simulink model "DivideNConquer"  (R2023a)
settings: Solver=VariableStepAuto  StartTime=0  StopTime=6012  MinStep=1e-2  RelTol=1e-3  AbsTol=1e-9
model workspace (MAT data in the model file):
  Cap = 4
  Grade = 0
  QHbatt = 70
  QLbatt = 40
  Trqmax = 400
  Vref = 650
values from neighbouring files (symbols this model uses):
  s = (id-1)*n_sim + 1    [LHSdesign.m]
undefined symbols (not defined in the file or in its folder): Qbatt, Vbatt
libraries: fl_lib x29, nesl_utility x15, sdl_lib x9, ee_lib x7, batteryecm_lib x1, autolibshared x1, slpidlib x1
(part 1 of 2)
settings Model: Creator=luiz4  LastModifiedBy=NUC04
settings SolverCC: MaxConsecutiveZCs=10000  MaxConsecutiveMinStep=12  ZeroCrossControl=EnableAll  ZeroCrossAlgorithm=Adaptive  EnableFixedStepZeroCrossing=on
settings OptimizationCC: ReuseModelBlockBuffer=off

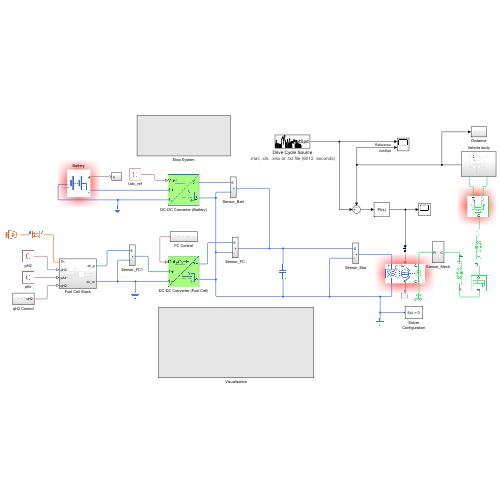
[thumbnail: Simulink's stored preview of the top-level diagram]
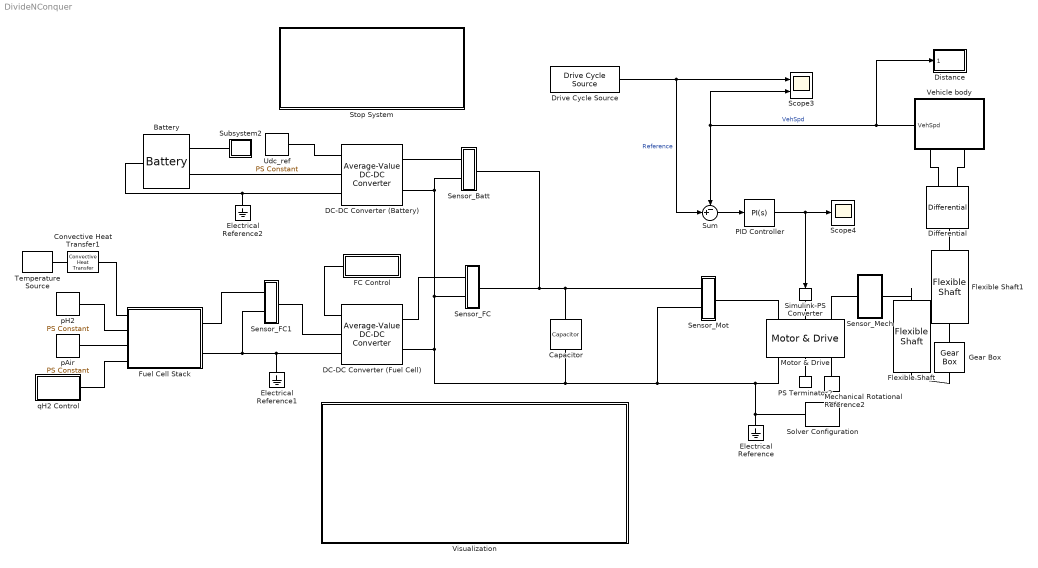
== system DivideNConquer ==
  Battery : batteryecm_lib/Battery  Vnom=Vbatt V  prm_dir=simscape.enum.battery.prm_dir.enabled  R1_dis=0.05 Ohm  R1_ch=0.05 Ohm  R1=0.05 Ohm  prm_AH=2  AH=Qbatt hr*A  V1=(4/5)*Vbatt V  AH1=0.5*Qbatt hr*A  prm_R2=1  R2=2000 Ohm  Tmeas=343.15 K  charge_measurement_port=simscape.enum.battery.enable.yes  prm_dyn=1  Rp1=0.005 Ohm  tau1=30 s  Rp2=0.005 Ohm  tau2=30 s  Rp3=0.005 Ohm  tau3=30 s  Rp4=0.005 Ohm  tau4=30 s  Rp5=0.005 Ohm  tau5=30 s  prm_fade=1  N_fade=100  AH_fade=45 hr*A  R1_fade=2.02 Ohm  R1_ch_fade=2.02 Ohm  V1_fade=10.35 V  prm_age=1  prm_age_OCV=1  OCV_age=0.9  SOC_age=60  Tmeas_age=298.15 K  delta_time_age_vec=[0] d  temperature_age_vec=[273] K  OCV_scaling_age=2.2134e6  OCV_offset_age=1.632e6  temp_exp_age=0.515833569 V  t_exp_age=0.75  Vnom_T2=12 V  R1_T2=2.2 Ohm  R1_T2_dis=2.2 Ohm  R1_T2_ch=2.2 Ohm  V1_T2=11.4 V  R2_T2=2200 Ohm  Rp1_T2=0.005 Ohm  tau1_T2=30 s  Rp2_T2=0.005 Ohm  tau2_T2=30 s  Rp3_T2=0.005 Ohm  tau3_T2=30 s  Rp4_T2=0.005 Ohm  tau4_T2=30 s  Rp5_T2=0.005 Ohm  tau5_T2=30 s  Tmeas2=273.15 K  thermal_port=simscape.enum.thermaleffects.omit  thermal_mass=30000 J/K  i_specify=off  i_priority=None  i=0 A  i_nominal_specify=off  i_nominal_unit=A  i_nominal_value=1  v_specify=on  v_priority=High  v=Vbatt V  v_nominal_specify=off  v_nominal_unit=V  v_nominal_value=1  charge_specify=on  charge_priority=High  charge=QHbatt*Qbatt/100 hr*A  charge_nominal_specify=off  charge_nominal_unit=A*hr  charge_nominal_value=1  num_cycles_specify=off  num_cycles_priority=High  num_cycles=0  num_cycles_nominal_specify=off  num_cycles_nominal_unit=1  num_cycles_nominal_value=1  temperature_specify=off  temperature_priority=High  temperature=298.15 K  temperature_nominal_specify=off  temperature_nominal_unit=K  temperature_nominal_value=1
      settings: LogSimulationData=on  InternalSimscapePortConfiguration="{\"Bottom\":[],\"Left\":[{\"id\":\"p\",\"label\":\"+\",\"type\":\"foundation.electrical.electrical\"},{\"id\":\"q\",\"label\":\"q\",\"type\":\"output\"}],\"Right\":[{\"id\":\"n\",\"label\":\"-\",\"type\":\"foundation.electrical.electrical\"}],\"Top\":[]}"
  Capacitor : fl_lib/Electrical/Electrical Elements/Capacitor  c=Cap F  r=1e-6 Ohm  g=0 1/Ohm  i_specify=off  i_priority=None  i=0 A  i_nominal_specify=off  i_nominal_unit=A  i_nominal_value=1  v_specify=off  v_priority=None  v=0 V  v_nominal_specify=off  v_nominal_unit=V  v_nominal_value=1  vc_specify=on  vc_priority=High  vc=0 V  vc_nominal_specify=on  vc_nominal_unit=V  vc_nominal_value=Vref
  Convective Heat Transfer1 : fl_lib/Thermal/Thermal Elements/Convective Heat Transfer  thermal_type=foundation.enum.constant_variable.constant  area=300 cm^2  heat_tr_coeff=75 W/(m^2 * K)  min_heat_tr_coeff=1e-3 W/(K*m^2)  T_specify=off  T_priority=None  T=0 K  T_nominal_specify=off  T_nominal_unit=K  T_nominal_value=1  Q_specify=off  Q_priority=None  Q=0 W  Q_nominal_specify=off  Q_nominal_unit=W  Q_nominal_value=1
  DC-DC Converter (Battery) : ee_lib/Semiconductors & Converters/Converters/Average-Value DC-DC Converter  control_option=ee.enum.converters.controlinput.voltage  converter_type=ee.enum.converters.dcdctype.boost  efficiency_option=ee.enum.converters.efficiency.constant  efficiency_fixed=90  i_vec=[0, 2, 5] A  efficiency_vec=[90, 95, 98]
      settings: LogSimulationData=on  InternalSimscapePortConfiguration="{\"Bottom\":[],\"Left\":[{\"id\":\"Vref\",\"label\":\"Vref\",\"type\":\"input\"},{\"id\":\"p1\",\"label\":\"1+\",\"type\":\"foundation.electrical.electrical\"},{\"id\":\"n1\",\"label\":\"1-\",\"type\":\"foundation.electrical.electrical\"}],\"Right\":[{\"id\":\"p2\",\"label\":\"2+\",\"type\":\"foundation.electrical.electrical\"},{\"id\":\"n2\",\"label\":\"2-\",\"type\":\"foundation.electrical.electrical\"}],\"Top\":[]}"
  DC-DC Converter (Fuel Cell) : ee_lib/Semiconductors & Converters/Converters/Average-Value DC-DC Converter  control_option=ee.enum.converters.controlinput.dutycycle  converter_type=ee.enum.converters.dcdctype.boost  efficiency_option=ee.enum.converters.efficiency.constant  efficiency_fixed=90  i_vec=[0, 2, 5] A  efficiency_vec=[90, 95, 98]
      settings: LogSimulationData=on  InternalSimscapePortConfiguration="{\"Bottom\":[],\"Left\":[{\"id\":\"DutyCycle\",\"label\":\"DutyCycle\",\"type\":\"input\"},{\"id\":\"p1\",\"label\":\"1+\",\"type\":\"foundation.electrical.electrical\"},{\"id\":\"n1\",\"label\":\"1-\",\"type\":\"foundation.electrical.electrical\"}],\"Right\":[{\"id\":\"p2\",\"label\":\"2+\",\"type\":\"foundation.electrical.electrical\"},{\"id\":\"n2\",\"label\":\"2-\",\"type\":\"foundation.electrical.electrical\"}],\"Top\":[]}"
  Differential : sdl_lib/Gears/Differential  driveshaft_location=sdl.enum.differential_orientation.right  cd_ratio=Rdiff  friction_model=sdl.enum.gear_friction.none  efficiency=[.85, .92]  temperature_TLU=[280, 300, 320] K  efficiency_ss_TLU=[.95, .9, .85]  efficiency_cd_TLU=[.95, .9, .85]  pwr_thr=[.001, .001] W  mu_visc=[0, 0] N*m*s/rad  model_inertia=simscape.enum.onoff.on  carrier_inertia=0.001 kg*m^2  planet_inertia=0.001 kg*m^2  thermal_mass=50 J/K  T_init=300 K
  Distance : Subsystem
  Drive Cycle Source : autolibshared/Drive Cycle Source  cycleVar=.mat, .xls, .xlsx or .txt file  wsVar=DriveCycle  fileVar=cycleMASTER.mat  tfinal="6012  seconds"  cycleRepeat=off  outAccPort=off  outGearPort=off  gearList=No gear data  t_wot1=5  xdot_woto=0  xdot_wot1=30  t_wot2=20  xdot_wot2=0  t_wotend=30  srcUnit=m/s  outUnit=m/s  srcAccUnit=m/s/s  outAccUnit=m/s^2  dt=0  aMode=1  faultOption=off  velBnd=2  velBndUnit=mph  inUnit=m/s  timeBnd=1  failOption=off  stopSim=off  maxFaultCnt=10  maxFaultTime=2  maxTotFaultTime=15  traceOption=off  dtTrace=1  traceWindow=10  lastDCname=Custom Data Set 1  lastOutUnit=mph  lastDT=0  lastTB=1  lastSB=2  forceCalcBound=off
  Electrical Reference : fl_lib/Electrical/Electrical Elements/Electrical Reference
  Electrical Reference1 : fl_lib/Electrical/Electrical Elements/Electrical Reference
  Electrical Reference2 : fl_lib/Electrical/Electrical Elements/Electrical Reference
  FC Control : Subsystem
  Flexible Shaft : sdl_lib/Couplings & Drives/Flexible Shaft  modelTorsion=true  modelTransverse=false  n_segments=1  parameterization=sdl.enum.shaftParameterization.StiffnessInertia  length=1 m  lengths=[1, .5, .25] m  shaft_stiffness=1e5 N*m/rad  shaft_inertia=0.1 kg*m^2  shaft_stiffnesses=[400000, 200000, 100000] N*m/rad  shaft_inertias=[.025, .02, .015] kg*m^2  eiIN=5e5 Pa*m^4  rhoaIN=19 kg/m  eiINs=[600000, 500000, 400000] Pa*m^4  rhoaINs=[20, 19, 18] kg/m  density=7.8e3 kg/m^3  shear_modulus=7.93e9 Pa  elastic_modulus=200e9 Pa  shaft_construction=sdl.enum.shaftConstruction.solid  diameter_outer=0.075 m  diameter_inner=0.05 m  diameter_outers=[.085, .075, .065] m  diameter_inners=[.055, .05, .045] m  damping_ratio=0.001  mu_visc_BF=[0, 0] N*m*s/rad  mu_visc=[0, 0] N*m*s/rad  initial_deflection=0 rad  initial_velocity=0 rpm  num_supports=sdl.enum.num_supports.two  z_support=[0, 1] m  boundaryB1=sdl.enum.shaftSupport.clamp  DrotB1_row=[1000, 1000] N*m*s/rad  DtransB1_row=[20000, -44000, -44000, 350000] N*s/m  DtransB1_w_mat=[20000, -44000, -44000, 350000; 10000, -25000, -25000, 140000; 5000, -10000, -10000, 20000] N*s/m  KrotB1_row=[10000, 10000] N*m/rad  KtransB1_row=[1000000, -200000, -300000, 5000000] N/m  KtransB1_w_mat=[1000000, -600000, -3500000, 8000000; 1000000, -200000, -3000000, 5000000; 1000000, -50000, -2500000, 3000000] N/m  boundaryI1=sdl.enum.shaftSupport.clamp  DrotI1_row=[1000, 1000] N*m*s/rad  DtransI1_row=[20000, -44000, -44000, 350000] N*s/m  DtransI1_w_mat=[20000, -44000, -44000, 350000; 10000, -25000, -25000, 140000; 5000, -10000, -10000, 20000] N*s/m  KrotI1_row=[10000, 10000] N*m/rad  KtransI1_row=[1000000, -200000, -300000, 5000000] N/m  KtransI1_w_mat=[1000000, -600000, -3500000, 8000000; 1000000, -200000, -3000000, 5000000; 1000000, -50000, -2500000, 3000000] N/m  boundaryI2=sdl.enum.shaftSupport.clamp  DrotI2_row=[1000, 1000] N*m*s/rad  DtransI2_row=[20000, -44000, -44000, 350000] N*s/m  DtransI2_w_mat=[20000, -44000, -44000, 350000; 10000, -25000, -25000, 140000; 5000, -10000, -10000, 20000] N*s/m  KrotI2_row=[10000, 10000] N*m/rad  KtransI2_row=[1000000, -200000, -300000, 5000000] N/m  KtransI2_w_mat=[1000000, -600000, -3500000, 8000000; 1000000, -200000, -3000000, 5000000; 1000000, -50000, -2500000, 3000000] N/m  boundaryF1=sdl.enum.shaftSupport.clamp  DrotF1_row=[1000, 1000] N*m*s/rad  DtransF1_row=[20000, -44000, -44000, 350000] N*s/m  DtransF1_w_mat=[20000, -44000, -44000, 350000; 10000, -25000, -25000, 140000; 5000, -10000, -10000, 20000] N*s/m  KrotF1_row=[10000, 10000] N*m/rad  KtransF1_row=[1000000, -200000, -300000, 5000000] N/m  KtransF1_w_mat=[1000000, -600000, -3500000, 8000000; 1000000, -200000, -3000000, 5000000; 1000000, -50000, -2500000, 3000000] N/m  bearing_speed=[200, 500, 1500] rpm  alpha=10 1/s  beta=1e-8 s  noDisk=sdl.enum.shaftDisks.none  zDisk=0.5 m  mDiskIN=2 kg  IdDiskIN=0.025 kg*m^2  IpDiskIN=0.050 kg*m^2  enable_static_unbalance=true  offsetMR=[.01, .01] kg*m  offsetMR_initialAngleIN=[0, pi] rad  offsetMassLocation=[.33, .67] m  enable_external_force=false  externalForce=[1, 2] N  externalForceHarmonic=[.5, 2]  externalLoadAngle=[pi / 2, 3 * pi / 4] rad  zExternalLoad=[.25, .75] m  AnalysisMethod=sdl.enum.bendingAnalysisMethod.LumpedMass  ModeInputMethod=sdl.enum.modeInputMethod.SimscapeDetermined  numModesIn=6  mode_speed_dependency=sdl.enum.mode_speed_dependency.Static  OmegaNom=5000 rpm  wMax=1e8 rpm  dz=0.01 m  userMode_w=[280, 644, 615, 1285] rad/s  userMode_w_mat=[257, 780, 580, 1560; 280, 644, 615, 1285; 294, 513, 636, 1020] rad/s  userMode_z=[0, .1, .2, .3, .4, .5, .6, .7, .8, .9, 1] m  userMode_shapeX=[.1648, .0086, -.2759, .0162; .1671, .0093, -.2231, .0133; .1691, .01, -.1689, .0102; .1707, .0105, -.1135, .007; .1717, .0108, -.057, .0035; .1721, .0109, 0, 0; .1717, .0108, .057, -.0035; .1707, .0105, .1135, -.007; .1691, .01, .1689, -.0102; .1671, .0093, .2231, -.0133; .1648, .0086, .2759, -.0162]  userMode_shapeX_mat=cat(3, [.1842, .0134, -.3072, .0272; .1863, .0152, -.2482, .0226; .1882, .0169, -.1878, .0176; .1897, .0182, -.1261, .0121; .1906, .019, -.0634, .0062; .191, .0193, 0, 0; .1906, .019, .0634, -.0062; .1897, .0182, .1261, -.0121; .1882, .0169, .1878, -.0176; .1863, .0152, .2482, -.0226; .1842, .0134, .3072, -.0272], [.1648, .0086, -.2759, .0162; .1671, .0093, -.2231, .0133; .1691, .01, -.1689, .0102; .1707, .0105, -.1135, .007; .1717, .0108, -.057, .0035; .1721, .0109, 0, 0; .1717, .0108, .057, -.0035; .1707, .0105, .1135, -.007; .1691, .01, .1689, -.0102; .1671, .0093, .2231, -.0133; .1648, .0086, .2759, -.0162], [.1291, .0046, -.2166, .0082; .131, .0048, -.1751, .0067; .1327, .005, -.1327, .0051; .1341, .0052, -.0891, .0035; .135, .0053, -.0448, .0017; .1353, .0053, 0, 0; .135, .0053, .0448, -.0017; .1341, .0052, .0891, -.0035; .1327, .005, .1327, -.0051; .131, .0048, .1751, -.0067; .1291, .0046, .2166, -.0082])  userMode_shapeY=[.1193, -.1784, -.1997, -.3348; .1209, -.1933, -.1615, -.2751; .1224, -.2068, -.1223, -.2119; .1235, -.2176, -.0821, -.1445; .1243, -.2245, -.0413, -.0734; .1246, -.2269, 0, 0; .1243, -.2245, .0413, .0734; .1235, -.2176, .0821, .1445; .1224, -.2068, .1223, .2119; .1209, -.1933, .1615, .2751; .1193, -.1784, .1997, .3348]  userMode_shapeY_mat=cat(3, [.0885, -.1625, -.1475, -.3301; .0895, -.1847, -.1192, -.2745; .0904, -.2048, -.0902, -.2141; .0911, -.2209, -.0606, -.1475; .0916, -.2313, -.0304, -.0754; .0917, -.2349, 0, 0; .0916, -.2313, .0304, .0754; .0911, -.2209, .0606, .1475; .0904, -.2048, .0902, .2141; .0895, -.1847, .1192, .2745; .0885, -.1625, .1475, .3301], [.1193, -.1784, -.1997, -.3348; .1209, -.1933, -.1615, -.2751; .1224, -.2068, -.1223, -.2119; .1235, -.2176, -.0821, -.1445; .1243, -.2245, -.0413, -.0734; .1246, -.2269, 0, 0; .1243, -.2245, .0413, .0734; .1235, -.2176, .0821, .1445; .1224, -.2068, .1223, .2119; .1209, -.1933, .1615, .2751; .1193, -.1784, .1997, .3348], [.1566, -.1901, -.2628, -.3377; .1589, -.1994, -.2125, -.2753; .161, -.2079, -.1609, -.2103; .1627, -.2146, -.1081, -.1424; .1638, -.219, -.0544, -.0719; .1642, -.2205, 0, 0; .1638, -.219, .0544, .0719; .1627, -.2146, .1081, .1424; .161, -.2079, .1609, .2103; .1589, -.1994, .2125, .2753; .1566, -.1901, .2628, .3377])  eta_lumped_nominal=1  etaDer_lumped_nominal=1  eta_modal_nominal=1  etaDer_modal_nominal=1
      settings: InternalSimscapePortConfiguration="{\"Bottom\":[],\"Left\":[{\"id\":\"B\",\"label\":\"B\",\"type\":\"foundation.mechanical.rotational.rotational\"}],\"Right\":[{\"id\":\"F\",\"label\":\"F\",\"type\":\"foundation.mechanical.rotational.rotational\"}],\"Top\":[]}"
  Flexible Shaft1 : sdl_lib/Couplings & Drives/Flexible Shaft  modelTorsion=true  modelTransverse=false  n_segments=1  parameterization=sdl.enum.shaftParameterization.StiffnessInertia  length=1 m  lengths=[1, .5, .25] m  shaft_stiffness=1e5 N*m/rad  shaft_inertia=0.1 kg*m^2  shaft_stiffnesses=[400000, 200000, 100000] N*m/rad  shaft_inertias=[.025, .02, .015] kg*m^2  eiIN=5e5 Pa*m^4  rhoaIN=19 kg/m  eiINs=[600000, 500000, 400000] Pa*m^4  rhoaINs=[20, 19, 18] kg/m  density=7.8e3 kg/m^3  shear_modulus=7.93e9 Pa  elastic_modulus=200e9 Pa  shaft_construction=sdl.enum.shaftConstruction.solid  diameter_outer=0.075 m  diameter_inner=0.05 m  diameter_outers=[.085, .075, .065] m  diameter_inners=[.055, .05, .045] m  damping_ratio=0.001  mu_visc_BF=[0, 0] N*m*s/rad  mu_visc=[0, 0] N*m*s/rad  initial_deflection=0 rad  initial_velocity=0 rpm  num_supports=sdl.enum.num_supports.two  z_support=[0, 1] m  boundaryB1=sdl.enum.shaftSupport.clamp  DrotB1_row=[1000, 1000] N*m*s/rad  DtransB1_row=[20000, -44000, -44000, 350000] N*s/m  DtransB1_w_mat=[20000, -44000, -44000, 350000; 10000, -25000, -25000, 140000; 5000, -10000, -10000, 20000] N*s/m  KrotB1_row=[10000, 10000] N*m/rad  KtransB1_row=[1000000, -200000, -300000, 5000000] N/m  KtransB1_w_mat=[1000000, -600000, -3500000, 8000000; 1000000, -200000, -3000000, 5000000; 1000000, -50000, -2500000, 3000000] N/m  boundaryI1=sdl.enum.shaftSupport.clamp  DrotI1_row=[1000, 1000] N*m*s/rad  DtransI1_row=[20000, -44000, -44000, 350000] N*s/m  DtransI1_w_mat=[20000, -44000, -44000, 350000; 10000, -25000, -25000, 140000; 5000, -10000, -10000, 20000] N*s/m  KrotI1_row=[10000, 10000] N*m/rad  KtransI1_row=[1000000, -200000, -300000, 5000000] N/m  KtransI1_w_mat=[1000000, -600000, -3500000, 8000000; 1000000, -200000, -3000000, 5000000; 1000000, -50000, -2500000, 3000000] N/m  boundaryI2=sdl.enum.shaftSupport.clamp  DrotI2_row=[1000, 1000] N*m*s/rad  DtransI2_row=[20000, -44000, -44000, 350000] N*s/m  DtransI2_w_mat=[20000, -44000, -44000, 350000; 10000, -25000, -25000, 140000; 5000, -10000, -10000, 20000] N*s/m  KrotI2_row=[10000, 10000] N*m/rad  KtransI2_row=[1000000, -200000, -300000, 5000000] N/m  KtransI2_w_mat=[1000000, -600000, -3500000, 8000000; 1000000, -200000, -3000000, 5000000; 1000000, -50000, -2500000, 3000000] N/m  boundaryF1=sdl.enum.shaftSupport.clamp  DrotF1_row=[1000, 1000] N*m*s/rad  DtransF1_row=[20000, -44000, -44000, 350000] N*s/m  DtransF1_w_mat=[20000, -44000, -44000, 350000; 10000, -25000, -25000, 140000; 5000, -10000, -10000, 20000] N*s/m  KrotF1_row=[10000, 10000] N*m/rad  KtransF1_row=[1000000, -200000, -300000, 5000000] N/m  KtransF1_w_mat=[1000000, -600000, -3500000, 8000000; 1000000, -200000, -3000000, 5000000; 1000000, -50000, -2500000, 3000000] N/m  bearing_speed=[200, 500, 1500] rpm  alpha=10 1/s  beta=1e-8 s  noDisk=sdl.enum.shaftDisks.none  zDisk=0.5 m  mDiskIN=2 kg  IdDiskIN=0.025 kg*m^2  IpDiskIN=0.050 kg*m^2  enable_static_unbalance=true  offsetMR=[.01, .01] kg*m  offsetMR_initialAngleIN=[0, pi] rad  offsetMassLocation=[.33, .67] m  enable_external_force=false  externalForce=[1, 2] N  externalForceHarmonic=[.5, 2]  externalLoadAngle=[pi / 2, 3 * pi / 4] rad  zExternalLoad=[.25, .75] m  AnalysisMethod=sdl.enum.bendingAnalysisMethod.LumpedMass  ModeInputMethod=sdl.enum.modeInputMethod.SimscapeDetermined  numModesIn=6  mode_speed_dependency=sdl.enum.mode_speed_dependency.Static  OmegaNom=5000 rpm  wMax=1e8 rpm  dz=0.01 m  userMode_w=[280, 644, 615, 1285] rad/s  userMode_w_mat=[257, 780, 580, 1560; 280, 644, 615, 1285; 294, 513, 636, 1020] rad/s  userMode_z=[0, .1, .2, .3, .4, .5, .6, .7, .8, .9, 1] m  userMode_shapeX=[.1648, .0086, -.2759, .0162; .1671, .0093, -.2231, .0133; .1691, .01, -.1689, .0102; .1707, .0105, -.1135, .007; .1717, .0108, -.057, .0035; .1721, .0109, 0, 0; .1717, .0108, .057, -.0035; .1707, .0105, .1135, -.007; .1691, .01, .1689, -.0102; .1671, .0093, .2231, -.0133; .1648, .0086, .2759, -.0162]  userMode_shapeX_mat=cat(3, [.1842, .0134, -.3072, .0272; .1863, .0152, -.2482, .0226; .1882, .0169, -.1878, .0176; .1897, .0182, -.1261, .0121; .1906, .019, -.0634, .0062; .191, .0193, 0, 0; .1906, .019, .0634, -.0062; .1897, .0182, .1261, -.0121; .1882, .0169, .1878, -.0176; .1863, .0152, .2482, -.0226; .1842, .0134, .3072, -.0272], [.1648, .0086, -.2759, .0162; .1671, .0093, -.2231, .0133; .1691, .01, -.1689, .0102; .1707, .0105, -.1135, .007; .1717, .0108, -.057, .0035; .1721, .0109, 0, 0; .1717, .0108, .057, -.0035; .1707, .0105, .1135, -.007; .1691, .01, .1689, -.0102; .1671, .0093, .2231, -.0133; .1648, .0086, .2759, -.0162], [.1291, .0046, -.2166, .0082; .131, .0048, -.1751, .0067; .1327, .005, -.1327, .0051; .1341, .0052, -.0891, .0035; .135, .0053, -.0448, .0017; .1353, .0053, 0, 0; .135, .0053, .0448, -.0017; .1341, .0052, .0891, -.0035; .1327, .005, .1327, -.0051; .131, .0048, .1751, -.0067; .1291, .0046, .2166, -.0082])  userMode_shapeY=[.1193, -.1784, -.1997, -.3348; .1209, -.1933, -.1615, -.2751; .1224, -.2068, -.1223, -.2119; .1235, -.2176, -.0821, -.1445; .1243, -.2245, -.0413, -.0734; .1246, -.2269, 0, 0; .1243, -.2245, .0413, .0734; .1235, -.2176, .0821, .1445; .1224, -.2068, .1223, .2119; .1209, -.1933, .1615, .2751; .1193, -.1784, .1997, .3348]  userMode_shapeY_mat=cat(3, [.0885, -.1625, -.1475, -.3301; .0895, -.1847, -.1192, -.2745; .0904, -.2048, -.0902, -.2141; .0911, -.2209, -.0606, -.1475; .0916, -.2313, -.0304, -.0754; .0917, -.2349, 0, 0; .0916, -.2313, .0304, .0754; .0911, -.2209, .0606, .1475; .0904, -.2048, .0902, .2141; .0895, -.1847, .1192, .2745; .0885, -.1625, .1475, .3301], [.1193, -.1784, -.1997, -.3348; .1209, -.1933, -.1615, -.2751; .1224, -.2068, -.1223, -.2119; .1235, -.2176, -.0821, -.1445; .1243, -.2245, -.0413, -.0734; .1246, -.2269, 0, 0; .1243, -.2245, .0413, .0734; .1235, -.2176, .0821, .1445; .1224, -.2068, .1223, .2119; .1209, -.1933, .1615, .2751; .1193, -.1784, .1997, .3348], [.1566, -.1901, -.2628, -.3377; .1589, -.1994, -.2125, -.2753; .161, -.2079, -.1609, -.2103; .1627, -.2146, -.1081, -.1424; .1638, -.219, -.0544, -.0719; .1642, -.2205, 0, 0; .1638, -.219, .0544, .0719; .1627, -.2146, .1081, .1424; .161, -.2079, .1609, .2103; .1589, -.1994, .2125, .2753; .1566, -.1901, .2628, .3377])  eta_lumped_nominal=1  etaDer_lumped_nominal=1  eta_modal_nominal=1  etaDer_modal_nominal=1
      settings: InternalSimscapePortConfiguration="{\"Bottom\":[],\"Left\":[{\"id\":\"B\",\"label\":\"B\",\"type\":\"foundation.mechanical.rotational.rotational\"}],\"Right\":[{\"id\":\"F\",\"label\":\"F\",\"type\":\"foundation.mechanical.rotational.rotational\"}],\"Top\":[]}"
  Fuel Cell Stack : Subsystem
  Gear Box : fl_lib/Mechanical/Mechanisms/Gear Box  ratio=5  t_in_specify=off  t_in_priority=None  t_in=0 N*m  t_in_nominal_specify=off  t_in_nominal_unit=N*m  t_in_nominal_value=1  t_out_specify=off  t_out_priority=None  t_out=0 N*m  t_out_nominal_specify=off  t_out_nominal_unit=N*m  t_out_nominal_value=1
  Mechanical Rotational Reference2 : fl_lib/Mechanical/Rotational Elements/Mechanical Rotational Reference
  Motor & Drive : sdl_lib/Engines & Motors/Motor & Drive  torque_max=Trqmax N*m  power_max=PMotmax kW  Tc=0.02 s  eff=80  w_eff=3750 rpm  T_eff=(7/8)*Trqmax N*m  thermal_port=simscape.enum.thermaleffects.omit  thermal_mass=100 J/K  temperature_specify=off  temperature_priority=High  temperature=300 K  temperature_nominal_specify=off  temperature_nominal_unit=K  temperature_nominal_value=1
      settings: InternalSimscapePortConfiguration="{\"Bottom\":[],\"Left\":[{\"id\":\"Vp\",\"label\":\"+\",\"type\":\"foundation.electrical.electrical\"},{\"id\":\"Tr\",\"label\":\"Tr\",\"type\":\"input\"},{\"id\":\"R\",\"label\":\"R\",\"type\":\"foundation.mechanical.rotational.rotational\"}],\"Right\":[{\"id\":\"Vm\",\"label\":\"-\",\"type\":\"foundation.electrical.electrical\"},{\"id\":\"Omega\",\"label\":\"w\",\"type\":\"output\"},{\"id\":\"C\",\"label\":\"C\",\"type\":\"foundation.mechanical.rotational.rotational\"}],\"Top\":[]}"
  PID Controller : slpidlib/PID Controller  Controller=PI  Form=Ideal  TimeDomain=Continuous-time  UseExternalTs=off  SampleTime=-1  IntegratorMethod=Forward Euler  FilterMethod=Forward Euler  ControllerParametersSource=internal  P=15  I=0.01  UseKiTs=off  D=100  N=100  UseFilter=on  TunerSelectOption=Transfer Function Based (PID Tuner App)  InitialConditionSource=internal  InitialConditionForIntegrator=0  InitialConditionForFilter=0  DifferentiatorICPrevScaledInput=0  ExternalReset=none  TrackingMode=off  Kt=1  LimitOutput=off  SatLimitsSource=internal  UpperSaturationLimit=inf  LowerSaturationLimit=-inf  LinearizeAsGain=on  AntiWindupMode=none  Kb=1  LimitIntegrator=off  UpperIntegratorSaturationLimit=inf  LowerIntegratorSaturationLimit=-inf  POutMin=[]  POutMax=[]  IOutMin=[]  IOutMax=[]  DOutMin=[]  DOutMax=[]  NOutMin=[]  NOutMax=[]  SumOutMin=[]  SumOutMax=[]  SaturationOutMin=[]  SaturationOutMax=[]  PParamMin=[]  PParamMax=[]  IParamMin=[]  IParamMax=[]  DParamMin=[]  DParamMax=[]  NParamMin=[]  NParamMax=[]  KbParamMin=[]  KbParamMax=[]  KtParamMin=[]  KtParamMax=[]  KbOutMin=[]  KbOutMax=[]  KtOutMin=[]  KtOutMax=[]  IntegratorOutMin=[]  IntegratorOutMax=[]  FilterOutMin=[]  FilterOutMax=[]  SumI1OutMin=[]  SumI1OutMax=[]  SumI2OutMin=[]  SumI2OutMax=[]  SumI3OutMin=[]  SumI3OutMax=[]  SumI4OutMin=[]  SumI4OutMax=[]  SumDOutMin=[]  SumDOutMax=[]  DifferentiatorOutMin=[]  DifferentiatorOutMax=[]  FilterDiffOutCoefMin=[]  FilterDiffOutCoefMax=[]  ReciprocalOutMin=[]  ReciprocalOutMax=[]  SumDenOutMin=[]  SumDenOutMax=[]  SumNumOutMin=[]  SumNumOutMax=[]  DivideOutMin=[]  DivideOutMax=[]  UdiffTsProdOutMin=[]  UdiffTsProdOutMax=[]  NTsProdOutMin=[]  NTsProdOutMax=[]  UintegralTsProdOutMin=[]  UintegralTsProdOutMax=[]  UngainTsProdOutMin=[]  UngainTsProdOutMax=[]  ClampingZeroOutDataTypeStr=Inherit: Inherit via back propagation  ClampingZeroOutMin=[]  ClampingZeroOutMax=[]  FilterDenConstantOutDataTypeStr=Inherit: Inherit via back propagation  FilterDenConstantOutMin=[]  FilterDenConstantOutMax=[]  PCopyOutDataTypeStr=Inherit: Inherit via back propagation  PCopyOutMin=[]  PCopyOutMax=[]  NCopyOutDataTypeStr=Inherit: Inherit via back propagation  NCopyOutMin=[]  NCopyOutMax=[]  IntegratorContinuousStateAttributes=''  IntegratorStateMustResolveToSignalObject=off  IntegratorRTWStateStorageClass=Auto  FilterContinuousStateAttributes=''  FilterStateMustResolveToSignalObject=off  FilterRTWStateStorageClass=Auto  ParallelPVariant=Passthrough  IdealPVariant=InternalParameters  IVariant=InternalParameters  DVariant=Disabled  IntegratorVariant=Continuous  SatVariant=Disabled  AWVariant=Passthrough  PCopyVariant=Disabled  TRVariant=Disabled  FdbkBlocksVariant=Forward  IdealPFdbkVariant=Disabled  SatFdbkVariant=Disabled  DerivativeFilterVariant=Disabled  NVariant=Disabled  NCopyVariant=Disabled_SignalSpec  FilterICVariant=Disabled  IntegratorICVariant=InternalICs  ExternalResetVariant=Disabled  TRSumVariant=Passthrough  SumFdbkVariant=Disabled  SumVariant=Sum_PI  TsampFilterVariant=InternalTs  TsampNgainVariant=Passthrough  TsampIntegralVariant=Disabled_SignalSpec  ExternalSaturationOutDataTypeStr=Inherit: Same as second input
  PS Terminator2 : fl_lib/Physical Signals/Sinks/PS Terminator
  Scope3 : Scope  NumInputPorts=2
  Scope4 : Scope
  Sensor_Batt : Subsystem
  Sensor_FC : Subsystem
  Sensor_FC1 : Subsystem
  Sensor_Mech : Subsystem
  Sensor_Mot : Subsystem
  Simulink-PS Converter : nesl_utility/Simulink-PS Converter  PhysicalDomain=network_engine_domain  SubClassName=ps_input  LeftPortType=input  RightPortType=output  PseudoPeriodic=off  Frequencies=[]  NoiseDistribution=none  NoiseParameters=[]  Unit=1  AffineConversion=off  FilteringAndDerivatives=filter  SimscapeFilterOrder=1  InputFilterTimeConstant=0.001  UdotUserProvided=0
  Solver Configuration : nesl_utility/Solver Configuration  PhysicalDomain=network_engine_domain  SubClassName=solver  LeftPortType=input  RightPortType=generic  Tones=[]  Harmonics=[]  SimulateNoise=off  Profile=off  UseLocalSampling=off  EnableSwitchedLinearOptims=on  FrequencyDomain=off  UseCCode=off  RelTol=0.001  AbsTol=1e-06  MinStep=1e-09  ToWorkspace=off  RevertToSquareIcSolve=off  NumHomotopyIterations=100  PhasorMode=off  PhasorModeNumHarmonics=1  ConsistencySolver=NEWTON_FTOL  IndexReductionMethod=DerivativeReplacement  DoDC=off  ResidualTolerance=1e-09  ConsistencyTolSource=GLOBAL  ConsistencyAbsTol=0.001  ConsistencyRelTol=0.001  ConsistencyTolFactor=0.001  UseLocalSolver=off  LocalSolverChoice=NE_BACKWARD_EULER_ADVANCER  ResolveIndetEquations=on  FunctionEvalNumThread=1  LocalSolverSampleTime=0.001  DoFixedCost=off  MaxNonlinIter=3  MaxModeIter=2  ComputeImpulses=off  ImpulseIterations=2  LinearAlgebra=auto  LinearAlgebraNumThread=0  EquationFormulation=NE_TIME_EF  DelaysMemoryBudget=1024  AutomaticFiltering=on  FilteringTimeConstant=0.001  PartitionStorageMethod=AS_NEEDED  PartitionMemoryBudget=1024  PartitionMethod=ROBUST
  Stop System : Subsystem
  Subsystem2 : Subsystem
  Sum : Sum  Inputs=-+|
  Temperature Source : fl_lib/Thermal/Thermal Sources/Temperature Source  temperature=293.15 K
  Udc_ref : fl_lib/Physical Signals/Sources/PS Constant  constant=Vref
  Vehicle body : Subsystem
      settings: PortSchema="{\"entries\":[{\"content\":{\"sides\":[{\"content\":{\"connectorIds\":[\"Out1\"]},\"type\":\"ConnectorPlacement.EquallySpacedRectSide\",\"uuid\":\"30e3ac76-7117-44d4-973a-6378fff16b47\"},{\"content\":{\"side\":\"RIGHT\"},\"type\":\"ConnectorPlacement.EquallySpacedRectSide\",\"uuid\":\"107753d6-a5ca-4ee3-aa53-d48c458c6d9d\"},{\"content\":{\"side\":\"TOP\"},\"type\":\"ConnectorPlacement.EquallySpacedRectSide\",\"uuid\":\"0a3e3c11-8cff-4941-9bcb-6ffb3d039700\"},{\"content\":{\"connectorIds\":[\"RConn1\",\"RConn2\"],\"side\":\"BOTTOM\"},\"type\":\"ConnectorPlacement.EquallySpacedRectSide\",\"uuid\":\"7585ecb7-2df2-4e77-9dfe-b3db33ebf8a5\"}]},\"type\":\"ConnectorPlacement.EquallySpacedConnector\",\"uuid\":\"e7d99235-5f65-4369-bb71-e85e0da50a7c\"}],\"packageUris\":[\"http://schema.mathworks.com/mf0/Connector/R2020b\"],\"version\":\"1.0\"}"
  Visualization : Subsystem
  pAir : fl_lib/Physical Signals/Sources/PS Constant  constant=1 bar
  pH2 : fl_lib/Physical Signals/Sources/PS Constant  constant=5.0 bar
  qH2 Control : Subsystem
  wires:
  PID Controller/1 -> Scope4/1, Simulink-PS Converter/1
  Sum/1 -> PID Controller/1
  Vehicle body/1(VehSpd) -> Distance/1(VehSpd), Sum/1, Scope3/2  "VehSpd"
  Drive Cycle Source/1 -> Sum/2, Scope3/1  "Reference"
  connections:
  Convective Heat Transfer1/LConn1 -- Fuel Cell Stack/LConn1
  DC-DC Converter (Fuel Cell)/RConn2 -- Capacitor/RConn1 -- Electrical Reference/LConn1 -- Solver Configuration/RConn1 -- Motor & Drive/RConn1 -- Sensor_Mot/LConn2 -- Sensor_Batt/LConn2 -- DC-DC Converter (Battery)/RConn2 -- Sensor_FC/LConn2
  Capacitor/LConn1 -- Sensor_Mot/LConn1 -- Sensor_Batt/RConn1 -- Sensor_FC/RConn1
  pAir/RConn1 -- Fuel Cell Stack/LConn3
  Temperature Source/LConn1 -- Convective Heat Transfer1/RConn1
  DC-DC Converter (Battery)/LConn2 -- Battery/LConn1
  Fuel Cell Stack/RConn2 -- Sensor_FC1/LConn2 -- Electrical Reference1/LConn1 -- DC-DC Converter (Fuel Cell)/LConn3
  DC-DC Converter (Battery)/RConn1 -- Sensor_Batt/LConn1
  Subsystem2/LConn1 -- Battery/LConn2
  DC-DC Converter (Fuel Cell)/RConn1 -- Sensor_FC/LConn1
  Battery/RConn1 -- Electrical Reference2/LConn1 -- DC-DC Converter (Battery)/LConn3
  pH2/RConn1 -- Fuel Cell Stack/LConn2
  Udc_ref/RConn1 -- DC-DC Converter (Battery)/LConn1
  Motor & Drive/RConn2 -- PS Terminator2/LConn1
  Flexible Shaft1/LConn1 -- Gear Box/RConn1
  Flexible Shaft1/RConn1 -- Differential/LConn1
  Motor & Drive/LConn2 -- Simulink-PS Converter/RConn1
  Gear Box/LConn1 -- Flexible Shaft/RConn1
  Flexible Shaft/LConn1 -- Sensor_Mech/RConn1
  Motor & Drive/LConn3 -- Sensor_Mech/LConn1
  Vehicle body/RConn1 -- Differential/RConn1
  Vehicle body/RConn2 -- Differential/RConn2
  Motor & Drive/LConn1 -- Sensor_Mot/RConn1
  FC Control/LConn1 -- DC-DC Converter (Fuel Cell)/LConn1
  qH2 Control/RConn1 -- Fuel Cell Stack/LConn4
  Mechanical Rotational Reference2/LConn1 -- Motor & Drive/RConn3
  Fuel Cell Stack/RConn1 -- Sensor_FC1/LConn1
  Sensor_FC1/RConn1 -- DC-DC Converter (Fuel Cell)/LConn2

== system DivideNConquer/Distance ==
  VehSpd : Inport
  Gain : Gain  Gain=1e-3
  Integrator : Integrator
  tag scope: Distance=global
  wires:
  VehSpd/1 -> Integrator/1
  Integrator/1 -> Gain/1
  Gain/1 -> [Distance]

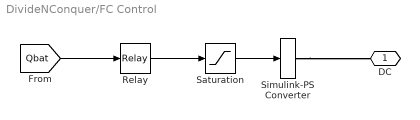
== system DivideNConquer/FC Control ==
  Relay : Relay  OnSwitchValue=QHbatt  OffSwitchValue=QLbatt
  Saturation : Saturate  UpperLimit=0.99  LowerLimit=0.05
  Simulink-PS Converter : nesl_utility/Simulink-PS Converter  PhysicalDomain=network_engine_domain  SubClassName=ps_input  LeftPortType=input  RightPortType=output  PseudoPeriodic=off  Frequencies=[]  NoiseDistribution=none  NoiseParameters=[]  Unit=1  AffineConversion=off  FilteringAndDerivatives=provide  SimscapeFilterOrder=1  InputFilterTimeConstant=0.001  UdotUserProvided=0
  DC : PMIOPort  Side=Left
  wires:
  Relay/1 -> Saturation/1
  Saturation/1 -> Simulink-PS Converter/1
  [Qbat] -> Relay/1
  connections:
  Simulink-PS Converter/RConn1 -- DC/RConn1

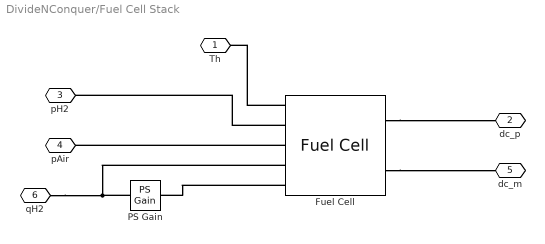
== system DivideNConquer/Fuel Cell Stack ==
  Fuel Cell : ee_lib/Sources/Fuel Cell  model_fidelity=ee.enum.fuelcell.fidelity.detailed  Eoc=65 V  A=0.23 V  ri=0.05 Ohm  i0=80 A  i_lim=200 A  N_cell=65  number_unit=10  pH2_nom=1.5e5 Pa  pO2_nom=1.0e5 Pa  xH2=99  xO2=21  xW=1  dyn=ee.enum.include.no  Rd=0.005 Ohm  tau=10 s  Tnom=293.15 K  thermal_mass=30000 J/K  iFC_specify=off  iFC_priority=None  iFC=0 A  iFC_nominal_specify=off  iFC_nominal_unit=A  iFC_nominal_value=1  vFC_specify=off  vFC_priority=None  vFC=0 V  vFC_nominal_specify=off  vFC_nominal_unit=V  vFC_nominal_value=1  temperature_specify=off  temperature_priority=High  temperature=293 K  temperature_nominal_specify=off  temperature_nominal_unit=K  temperature_nominal_value=1
      settings: InternalSimscapePortConfiguration="{\"Bottom\":[],\"Left\":[{\"id\":\"H\",\"label\":\"H\",\"type\":\"foundation.thermal.thermal\"},{\"id\":\"pfuel\",\"label\":\"pfuel\",\"type\":\"input\"},{\"id\":\"pair\",\"label\":\"pair\",\"type\":\"input\"},{\"id\":\"qfuel\",\"label\":\"qfuel\",\"type\":\"input\"},{\"id\":\"qair\",\"label\":\"qair\",\"type\":\"input\"}],\"Right\":[{\"id\":\"p\",\"label\":\"+\",\"type\":\"foundation.electrical.electrical\"},{\"id\":\"n\",\"label\":\"-\",\"type\":\"foundation.electrical.electrical\"}],\"Top\":[]}"
  PS Gain : fl_lib/Physical Signals/Functions/PS Gain  gain=3
  Th : PMIOPort  Side=Left
  dc_p : PMIOPort  Port=2  Side=Right
  pH2 : PMIOPort  Port=3  Side=Left
  pAir : PMIOPort  Port=4  Side=Left
  dc_m : PMIOPort  Port=5  Side=Right
  qH2 : PMIOPort  Port=6  Side=Left
  connections:
  Fuel Cell/RConn2 -- dc_m/RConn1
  Fuel Cell/LConn2 -- pH2/RConn1
  Fuel Cell/LConn5 -- PS Gain/RConn1
  PS Gain/LConn1 -- Fuel Cell/LConn4 -- qH2/RConn1
  Fuel Cell/LConn3 -- pAir/RConn1
  Fuel Cell/LConn1 -- Th/RConn1
  Fuel Cell/RConn1 -- dc_p/RConn1

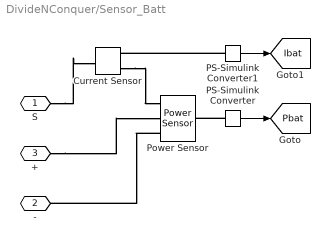
== system DivideNConquer/Sensor_Batt ==
  Current Sensor : fl_lib/Electrical/Electrical Sensors/Current Sensor
  PS-Simulink Converter : nesl_utility/PS-Simulink Converter  PhysicalDomain=network_engine_domain  SubClassName=ps_output  LeftPortType=input  RightPortType=output  PseudoPeriodic=off  Frequencies=[]  VectorFormat=1-D array  Unit=kW  AffineConversion=off
  PS-Simulink Converter1 : nesl_utility/PS-Simulink Converter  PhysicalDomain=network_engine_domain  SubClassName=ps_output  LeftPortType=input  RightPortType=output  PseudoPeriodic=off  Frequencies=[]  VectorFormat=1-D array  Unit=A  AffineConversion=off
  Power Sensor : ee_lib/Sensors & Transducers/Power Sensor  measurement_type=1  averaging_period=1e-4 s
  S : PMIOPort  Side=Left
  - : PMIOPort  Port=2  Side=Left
  + : PMIOPort  Port=3  Side=Right
  tag scope: Ibat=global, Pbat=global
  wires:
  PS-Simulink Converter/1 -> [Pbat]
  PS-Simulink Converter1/1 -> [Ibat]
  connections:
  +/RConn1 -- Power Sensor/LConn2
  Power Sensor/LConn3 -- -/RConn1
  PS-Simulink Converter/LConn1 -- Power Sensor/RConn1
  Current Sensor/RConn2 -- Power Sensor/LConn1
  S/RConn1 -- Current Sensor/LConn1
  PS-Simulink Converter1/LConn1 -- Current Sensor/RConn1

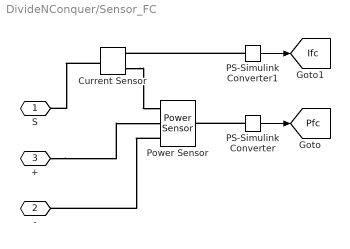
== system DivideNConquer/Sensor_FC ==
  Current Sensor : fl_lib/Electrical/Electrical Sensors/Current Sensor
  PS-Simulink Converter : nesl_utility/PS-Simulink Converter  PhysicalDomain=network_engine_domain  SubClassName=ps_output  LeftPortType=input  RightPortType=output  PseudoPeriodic=off  Frequencies=[]  VectorFormat=1-D array  Unit=kW  AffineConversion=off
  PS-Simulink Converter1 : nesl_utility/PS-Simulink Converter  PhysicalDomain=network_engine_domain  SubClassName=ps_output  LeftPortType=input  RightPortType=output  PseudoPeriodic=off  Frequencies=[]  VectorFormat=1-D array  Unit=A  AffineConversion=off
  Power Sensor : ee_lib/Sensors & Transducers/Power Sensor  measurement_type=1  averaging_period=1e-4 s
  S : PMIOPort  Side=Left
  - : PMIOPort  Port=2  Side=Left
  + : PMIOPort  Port=3  Side=Right
  tag scope: Ifc=global, Pfc=global
  wires:
  PS-Simulink Converter/1 -> [Pfc]
  PS-Simulink Converter1/1 -> [Ifc]
  connections:
  +/RConn1 -- Power Sensor/LConn2
  Power Sensor/LConn3 -- -/RConn1
  PS-Simulink Converter/LConn1 -- Power Sensor/RConn1
  PS-Simulink Converter1/LConn1 -- Current Sensor/RConn1
  Current Sensor/LConn1 -- S/RConn1
  Current Sensor/RConn2 -- Power Sensor/LConn1

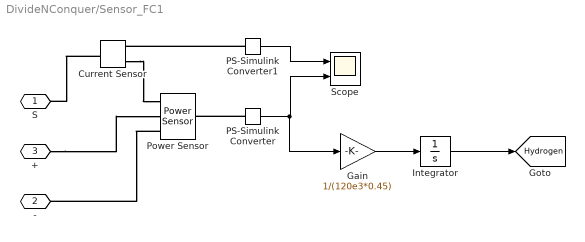
== system DivideNConquer/Sensor_FC1 ==
  Current Sensor : fl_lib/Electrical/Electrical Sensors/Current Sensor
  Gain : Gain  Gain=1/(120e3*0.45)
  Integrator : Integrator
  PS-Simulink Converter : nesl_utility/PS-Simulink Converter  PhysicalDomain=network_engine_domain  SubClassName=ps_output  LeftPortType=input  RightPortType=output  PseudoPeriodic=off  Frequencies=[]  VectorFormat=1-D array  Unit=kW  AffineConversion=off
  PS-Simulink Converter1 : nesl_utility/PS-Simulink Converter  PhysicalDomain=network_engine_domain  SubClassName=ps_output  LeftPortType=input  RightPortType=output  PseudoPeriodic=off  Frequencies=[]  VectorFormat=1-D array  Unit=A  AffineConversion=off
  Power Sensor : ee_lib/Sensors & Transducers/Power Sensor  measurement_type=1  averaging_period=1e-4 s
  Scope : Scope  NumInputPorts=2
  S : PMIOPort  Side=Left
  - : PMIOPort  Port=2  Side=Left
  + : PMIOPort  Port=3  Side=Right
  tag scope: Hydrogen=global
  wires:
  PS-Simulink Converter/1 -> Gain/1, Scope/2
  PS-Simulink Converter1/1 -> Scope/1
  Gain/1 -> Integrator/1
  Integrator/1 -> [Hydrogen]
  connections:
  +/RConn1 -- Power Sensor/LConn2
  Power Sensor/LConn3 -- -/RConn1
  PS-Simulink Converter/LConn1 -- Power Sensor/RConn1
  PS-Simulink Converter1/LConn1 -- Current Sensor/RConn1
  Current Sensor/LConn1 -- S/RConn1
  Current Sensor/RConn2 -- Power Sensor/LConn1

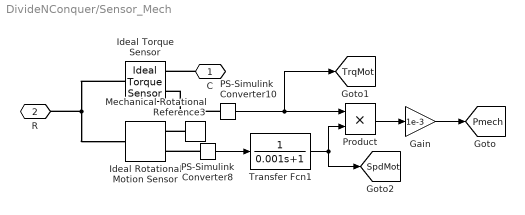
== system DivideNConquer/Sensor_Mech ==
  Gain : Gain  Gain=1e-3
  Ideal Rotational Motion Sensor : fl_lib/Mechanical/Mechanical Sensors/Ideal Rotational Motion Sensor  reference=foundation.enum.MeasurementReference.difference  acceleration_port=false  velocity_port=true  position_port=false  wrap_angle=false  offset=0 rad
      settings: InternalSimscapePortConfiguration="{\"Bottom\":[],\"Left\":[{\"id\":\"R\",\"label\":\"R\",\"type\":\"foundation.mechanical.rotational.rotational\"}],\"Right\":[{\"id\":\"C\",\"label\":\"C\",\"type\":\"foundation.mechanical.rotational.rotational\"},{\"id\":\"W\",\"label\":\"W\",\"type\":\"output\"}],\"Top\":[]}"
  Ideal Torque Sensor : fl_lib/Mechanical/Mechanical Sensors/Ideal Torque Sensor
  Mechanical Rotational Reference3 : fl_lib/Mechanical/Rotational Elements/Mechanical Rotational Reference
  PS-Simulink Converter10 : nesl_utility/PS-Simulink Converter  PhysicalDomain=network_engine_domain  SubClassName=ps_output  LeftPortType=input  RightPortType=output  PseudoPeriodic=off  Frequencies=[]  VectorFormat=inherit  Unit=inherit  AffineConversion=off
  PS-Simulink Converter8 : nesl_utility/PS-Simulink Converter  PhysicalDomain=network_engine_domain  SubClassName=ps_output  LeftPortType=input  RightPortType=output  PseudoPeriodic=off  Frequencies=[]  VectorFormat=inherit  Unit=inherit  AffineConversion=off
  Product : Product
  Transfer Fcn1 : TransferFcn  Denominator=[0.001 1]
  C : PMIOPort  Side=Right
  R : PMIOPort  Port=2  Side=Left
  tag scope: Pmech=global, SpdMot=global, TrqMot=global
  wires:
  PS-Simulink Converter10/1 -> [TrqMot], Product/1
  Transfer Fcn1/1 -> Product/2, [SpdMot]
  PS-Simulink Converter8/1 -> Transfer Fcn1/1
  Product/1 -> Gain/1
  Gain/1 -> [Pmech]
  connections:
  PS-Simulink Converter8/LConn1 -- Ideal Rotational Motion Sensor/RConn2
  PS-Simulink Converter10/LConn1 -- Ideal Torque Sensor/RConn2
  Mechanical Rotational Reference3/LConn1 -- Ideal Rotational Motion Sensor/RConn1
  Ideal Torque Sensor/LConn1 -- Ideal Rotational Motion Sensor/LConn1 -- R/RConn1
  C/RConn1 -- Ideal Torque Sensor/RConn1

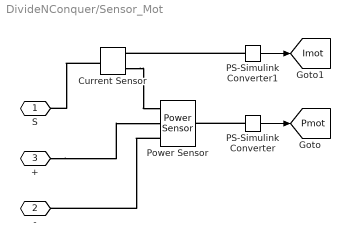
== system DivideNConquer/Sensor_Mot ==
  Current Sensor : fl_lib/Electrical/Electrical Sensors/Current Sensor
  PS-Simulink Converter : nesl_utility/PS-Simulink Converter  PhysicalDomain=network_engine_domain  SubClassName=ps_output  LeftPortType=input  RightPortType=output  PseudoPeriodic=off  Frequencies=[]  VectorFormat=1-D array  Unit=kW  AffineConversion=off
  PS-Simulink Converter1 : nesl_utility/PS-Simulink Converter  PhysicalDomain=network_engine_domain  SubClassName=ps_output  LeftPortType=input  RightPortType=output  PseudoPeriodic=off  Frequencies=[]  VectorFormat=1-D array  Unit=A  AffineConversion=off
  Power Sensor : ee_lib/Sensors & Transducers/Power Sensor  measurement_type=1  averaging_period=1e-4 s
  S : PMIOPort  Side=Left
  - : PMIOPort  Port=2  Side=Left
  + : PMIOPort  Port=3  Side=Right
  tag scope: Imot=global, Pmot=global
  wires:
  PS-Simulink Converter/1 -> [Pmot]
  PS-Simulink Converter1/1 -> [Imot]
  connections:
  +/RConn1 -- Power Sensor/LConn2
  Power Sensor/LConn3 -- -/RConn1
  PS-Simulink Converter/LConn1 -- Power Sensor/RConn1
  PS-Simulink Converter1/LConn1 -- Current Sensor/RConn1
  Current Sensor/LConn1 -- S/RConn1
  Current Sensor/RConn2 -- Power Sensor/LConn1

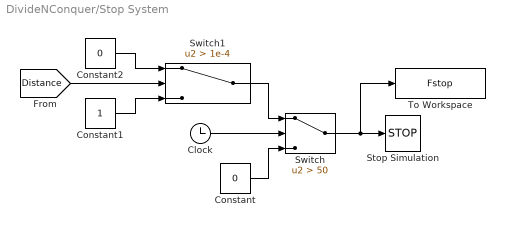
== system DivideNConquer/Stop System ==
  Clock : Clock
  Constant : Constant  Value=0
  Constant1 : Constant
  Constant2 : Constant  Value=0
  Stop Simulation : Stop
  Switch : Switch  Criteria=u2 > Threshold  Threshold=50  SaturateOnIntegerOverflow=off  InputSameDT=off
  Switch1 : Switch  Criteria=u2 > Threshold  Threshold=1e-4  SaturateOnIntegerOverflow=off  InputSameDT=off
  To Workspace : ToWorkspace  VariableName=Fstop  SampleTime=-1
      settings: MaxDataPoints=1  Save2DSignal=2-D array (concatenate along first dimension)
  wires:
  Switch/1 -> To Workspace/1, Stop Simulation/1
  Clock/1 -> Switch/2
  [Distance] -> Switch1/2
  Switch1/1 -> Switch/1
  Constant2/1 -> Switch1/1
  Constant1/1 -> Switch1/3
  Constant/1 -> Switch/3

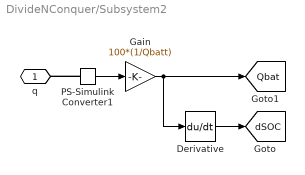
== system DivideNConquer/Subsystem2 ==
  Derivative : Derivative
  Gain : Gain  Gain=100*(1/Qbatt)
  PS-Simulink Converter1 : nesl_utility/PS-Simulink Converter  PhysicalDomain=network_engine_domain  SubClassName=ps_output  LeftPortType=input  RightPortType=output  PseudoPeriodic=off  Frequencies=[]  VectorFormat=1-D array  Unit=A*hr  AffineConversion=off
  q : PMIOPort  Side=Left
  tag scope: Qbat=global, dSOC=global
  wires:
  PS-Simulink Converter1/1 -> Gain/1
  Gain/1 -> Derivative/1, [Qbat]
  Derivative/1 -> [dSOC]
  connections:
  PS-Simulink Converter1/LConn1 -- q/RConn1

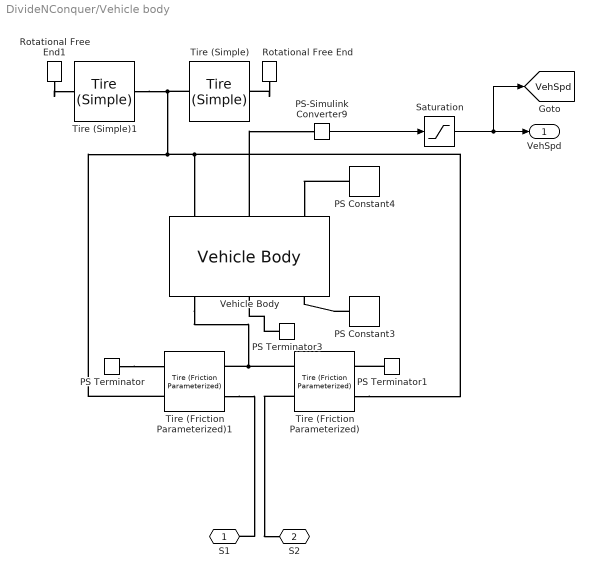
== system DivideNConquer/Vehicle body ==
  PS Constant3 : fl_lib/Physical Signals/Sources/PS Constant  constant=Grade rad
  PS Constant4 : fl_lib/Physical Signals/Sources/PS Constant  constant=0
  PS Terminator : fl_lib/Physical Signals/Sinks/PS Terminator
  PS Terminator1 : fl_lib/Physical Signals/Sinks/PS Terminator
  PS Terminator3 : fl_lib/Physical Signals/Sinks/PS Terminator
  PS-Simulink Converter9 : nesl_utility/PS-Simulink Converter  PhysicalDomain=network_engine_domain  SubClassName=ps_output  LeftPortType=input  RightPortType=output  PseudoPeriodic=off  Frequencies=[]  VectorFormat=inherit  Unit=inherit  AffineConversion=off
  Rotational Free End : fl_lib/Mechanical/Rotational Elements/Rotational Free End  w_specify=off  w_priority=None  w=0 rad/s  w_nominal_specify=off  w_nominal_unit=rad/s  w_nominal_value=1
  Rotational Free End1 : fl_lib/Mechanical/Rotational Elements/Rotational Free End  w_specify=off  w_priority=None  w=0 rad/s  w_nominal_specify=off  w_nominal_unit=rad/s  w_nominal_value=1
  Saturation : Saturate  UpperLimit=inf  LowerLimit=0  ZeroCross=off
  Tire (Friction Parameterized) : sdl_lib/Tires & Vehicles/Tire (Friction Parameterized)  r_tire=Rwheel m  slip_output=sdl.enum.SlipOutput.Relative  friction_model=sdl.enum.friction_model_var.fixed  mu_static=0.90  mu_kinetic=0.70  slip_vector=[0, .02, .06, .15, .6, 1] rad/s  mu_kinetic_vector=[.89, .88, .8, .75, .7, .7]  interp_method=simscape.enum.interpolation.linear  extrap_method=simscape.enum.extrapolation.linear  model_compliance=sdl.enum.compliance.off  stiffness=1e6 N/m  damping=1000 N*s/m  model_inertia=sdl.enum.model_inertia.on  tire_inertia=0.8 kg*m^2  initial_velocity=0 rad/s  model_resistance=simscape.enum.onoff.off  resistance_model=sdl.enum.RollingResistance.Constant  coeff=0.015  p_tire=250e3 Pa  alpha=-0.003  beta=0.97  coeff_a=84e-4  coeff_b=6.2e-4 s/m  coeff_c=1.6e-4 s^2/m^2  v_thr=0.001 m/s  v_tol=0.01 m/s  F_min=10 N  initial_traction_state=sdl.enum.tireIC.traction
      settings: InternalSimscapePortConfiguration="{\"Bottom\":[],\"Left\":[{\"id\":\"N\",\"label\":\"N\",\"type\":\"input\"},{\"id\":\"A\",\"label\":\"A\",\"type\":\"foundation.mechanical.rotational.rotational\"}],\"Right\":[{\"id\":\"Srel\",\"label\":\"S\",\"type\":\"output\"},{\"id\":\"H\",\"label\":\"H\",\"type\":\"foundation.mechanical.translational.translational\"}],\"Top\":[]}"
  Tire (Friction Parameterized)1 : sdl_lib/Tires & Vehicles/Tire (Friction Parameterized)  r_tire=Rwheel m  slip_output=sdl.enum.SlipOutput.Relative  friction_model=sdl.enum.friction_model_var.fixed  mu_static=0.90  mu_kinetic=0.70  slip_vector=[0, .02, .06, .15, .6, 1] rad/s  mu_kinetic_vector=[.89, .88, .8, .75, .7, .7]  interp_method=simscape.enum.interpolation.linear  extrap_method=simscape.enum.extrapolation.linear  model_compliance=sdl.enum.compliance.off  stiffness=1e6 N/m  damping=1000 N*s/m  model_inertia=sdl.enum.model_inertia.on  tire_inertia=0.8 kg*m^2  initial_velocity=0 rad/s  model_resistance=simscape.enum.onoff.off  resistance_model=sdl.enum.RollingResistance.Constant  coeff=0.015  p_tire=250e3 Pa  alpha=-0.003  beta=0.97  coeff_a=84e-4  coeff_b=6.2e-4 s/m  coeff_c=1.6e-4 s^2/m^2  v_thr=0.001 m/s  v_tol=0.01 m/s  F_min=10 N  initial_traction_state=sdl.enum.tireIC.traction
      settings: InternalSimscapePortConfiguration="{\"Bottom\":[],\"Left\":[{\"id\":\"N\",\"label\":\"N\",\"type\":\"input\"},{\"id\":\"A\",\"label\":\"A\",\"type\":\"foundation.mechanical.rotational.rotational\"}],\"Right\":[{\"id\":\"Srel\",\"label\":\"S\",\"type\":\"output\"},{\"id\":\"H\",\"label\":\"H\",\"type\":\"foundation.mechanical.translational.translational\"}],\"Top\":[]}"
  Tire (Simple) : sdl_lib/Tires & Vehicles/Tire (Simple)  r_tire=Rwheel m  model_compliance=sdl.enum.compliance.off  stiffness=1e6 N/m  damping=1000 N*s/m  model_inertia=sdl.enum.model_inertia.on  tire_inertia=0.8 kg*m^2  initial_velocity=0 rad/s
      settings: InternalSimscapePortConfiguration="{\"Bottom\":[],\"Left\":[{\"id\":\"A\",\"label\":\"A\",\"type\":\"foundation.mechanical.rotational.rotational\"}],\"Right\":[{\"id\":\"H\",\"label\":\"H\",\"type\":\"foundation.mechanical.translational.translational\"}],\"Top\":[]}"
  Tire (Simple)1 : sdl_lib/Tires & Vehicles/Tire (Simple)  r_tire=Rwheel m  model_compliance=sdl.enum.compliance.off  stiffness=1e6 N/m  damping=1000 N*s/m  model_inertia=sdl.enum.model_inertia.on  tire_inertia=0.8 kg*m^2  initial_velocity=0 rad/s
      settings: InternalSimscapePortConfiguration="{\"Bottom\":[],\"Left\":[{\"id\":\"A\",\"label\":\"A\",\"type\":\"foundation.mechanical.rotational.rotational\"}],\"Right\":[{\"id\":\"H\",\"label\":\"H\",\"type\":\"foundation.mechanical.translational.translational\"}],\"Top\":[]}"
  Vehicle Body : sdl_lib/Tires & Vehicles/Vehicle Body  mass=Mvehicle kg  n_w=2  x_f=1.358 m  x_r=1.552 m  y_c=0.5 m  mass_var=simscape.enum.onoff.off  g=9.81 m/s^2  liftoff_warning=simscape.enum.onoff.off  area=2.7636 m^2  Cd=0.4  rho=1.18 kg/m^3  model_pitch=simscape.enum.onoff.off  inertia=4000 kg*m^2  suspension_model=sdl.enum.linearTLU.linear  k_f=1e4 N/m  b_f=1e4 N*s/m  k_r=1e4 N/m  b_r=1e4 N*s/m  k_f_TLU=[-2000, -1000, 0, 1000, 2000] N  x_f_TLU=[-.4, -.2, 0, .2, .4] m  b_f_TLU=[-200, -100, 0, 100, 200] N  v_f_TLU=[-4, -2, 0, 2, 4] m/s  k_r_TLU=[-2000, -1000, 0, 1000, 2000] N  x_r_TLU=[-.4, -.2, 0, .2, .4] m  b_r_TLU=[-200, -100, 0, 100, 200] N  v_r_TLU=[-4, -2, 0, 2, 4] m/s  interp_method=simscape.enum.interpolation.linear  extrap_method=simscape.enum.extrapolation.linear  model_hardstop=simscape.enum.onoff.off  upper_bound_f=.25 m  lower_bound_f=-.25 m  stop_k_f=1e6 N/m  stop_b_f=150 N*s/m  upper_bound_r=.25 m  lower_bound_r=-.25 m  stop_k_r=1e6 N/m  stop_b_r=150 N*s/m  initial_pitch=0 rad  initial_pitch_rate=0 rad/s  v_specify=off  v_priority=High  v=0 m/s  v_nominal_specify=off  v_nominal_unit=m/s  v_nominal_value=1
  S1 : PMIOPort  Side=Right
  S2 : PMIOPort  Port=2  Side=Right
  VehSpd : Outport
  tag scope: VehSpd=global
  wires:
  PS-Simulink Converter9/1 -> Saturation/1
  Saturation/1 -> [VehSpd], VehSpd/1
  connections:
  Rotational Free End/LConn1 -- Tire (Simple)/LConn1
  Tire (Friction Parameterized)/LConn1 -- Vehicle Body/RConn1 -- Tire (Friction Parameterized)1/LConn1
  Tire (Simple)/RConn1 -- Tire (Simple)1/RConn1 -- Tire (Friction Parameterized)/RConn2 -- Vehicle Body/LConn1 -- Tire (Friction Parameterized)1/RConn2
  PS Terminator3/LConn1 -- Vehicle Body/RConn2
  Vehicle Body/LConn2 -- PS-Simulink Converter9/LConn1
  PS Terminator/LConn1 -- Tire (Friction Parameterized)1/RConn1
  PS Constant4/RConn1 -- Vehicle Body/LConn3
  PS Terminator1/LConn1 -- Tire (Friction Parameterized)/RConn1
  PS Constant3/RConn1 -- Vehicle Body/RConn3
  Rotational Free End1/LConn1 -- Tire (Simple)1/LConn1
  Tire (Friction Parameterized)1/LConn2 -- S1/RConn1
  Tire (Friction Parameterized)/LConn2 -- S2/RConn1
